simulink model "CR_quarter_car_NL"  (R2025b)
settings: Solver=VariableStepAuto  StartTime=0.0  StopTime=20  RelTol=1e-9
values from neighbouring files (symbols this model uses):
  omega_n1 = 80    [A_quarter_car_parameters.m]    (also in A_uncertain_Plant.m = parameters.omega_n1; Incert_plant.m; LQG.m; LQG_pt2.m)
  tau_1 = 0.005    [A_quarter_car_parameters.m]    (also in LQG.m; LQG_pt2.m; LQG_pt2.mat; Lin_model.m)
  tau_2 = 0.010    (= 0.01)    [A_quarter_car_parameters.m]    (also in LQG.m; LQG_pt2.m; LQG_pt2.mat; Lin_model.m)
  tau_a = 0.025    [A_quarter_car_parameters.m]    (also in A_uncertain_Plant.m = parameters.tau_a; Incert_plant.m; LQG.m; LQG_pt2.m)
  x0_delta_s = 0    [A_quarter_car_parameters.m]    (also in quarter_car_parameters.m)
  x0_delta_t = 0    [A_quarter_car_parameters.m]    (also in quarter_car_parameters.m)
  x0_zs_dot = 0    [A_quarter_car_parameters.m]    (also in quarter_car_parameters.m)
  x0_zu_dot = 0    [A_quarter_car_parameters.m]    (also in quarter_car_parameters.m)
  zeta_1 = 0.7    [A_quarter_car_parameters.m]    (also in A_uncertain_Plant.m = parameters.zeta_1; Incert_plant.m; LQG.m; LQG_pt2.m)
libraries: simulink x12, cstblocks x2
settings Model: Creator=roly2  LastModifiedBy=ettor

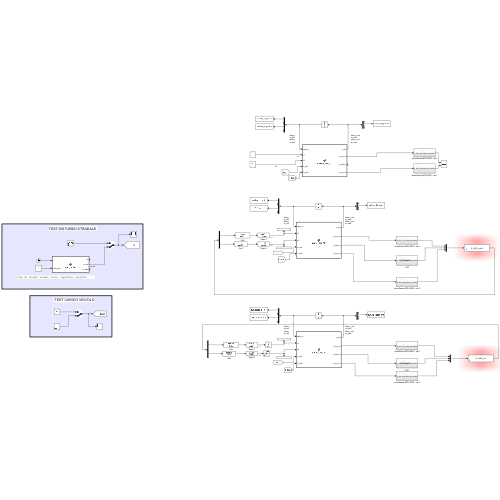
[thumbnail: Simulink's stored preview of the top-level diagram]
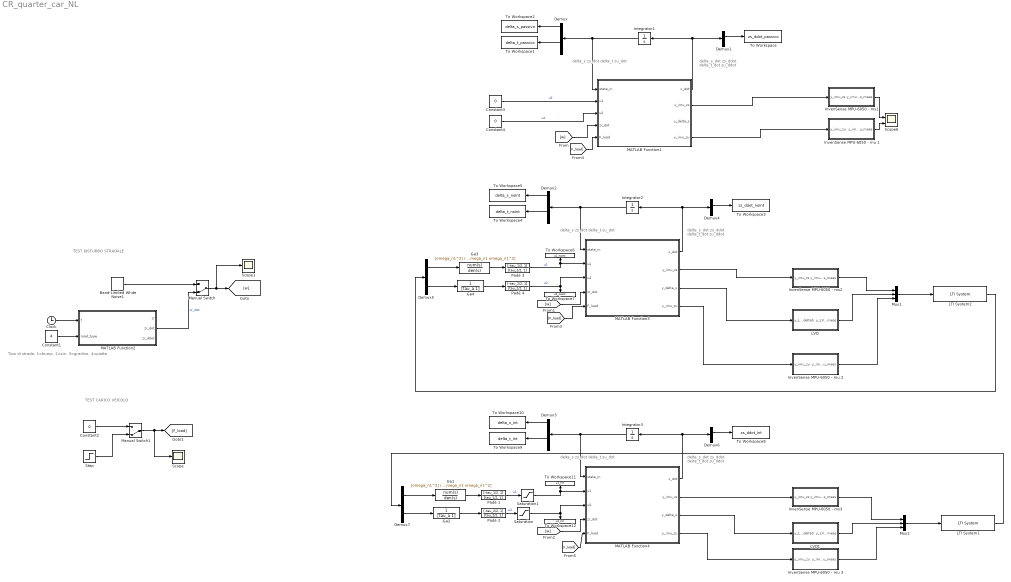
== system CR_quarter_car_NL ==
  note: TEST CARICO VEICOLO
  note: Tipo di strada: 1=bump, 2=sin, 3=gradino, 4=piatta
  note: delta_s_dot
      | zs_ddot
      | delta_t_dot
      | zu_ddot
  note: delta_s
      | zs_dot
      | delta_t
      | zu_dot
  note: delta_s
      | zs_dot
      | delta_t
      | zu_dot
  note: delta_s_dot
      | zs_ddot
      | delta_t_dot
      | zu_ddot
  note: delta_s_dot
      | zs_ddot
      | delta_t_dot
      | zu_ddot
  note: delta_s
      | zs_dot
      | delta_t
      | zu_dot
  note: TEST DISTURBO STRADALE
  Band-Limited White Noise1 : simulink/Sources/Band-Limited White Noise  Cov=[0.0001]  Ts=0.01  seed=[23341]
  Clock : Clock
  Constant1 : Constant  Value=4
  Constant2 : Constant  Value=0
  Constant3 : Constant  Value=0
  Constant4 : Constant  Value=0
  Demux{,1..4,6} (6 alike) : Demux
  Demux5 : Demux  Outputs=2
  Demux7 : Demux  Outputs=2
  Ga1 : TransferFcn  Numerator=[omega_n1^2]  Denominator=[1 2*zeta_1*omega_n1 omega_n1^2]
  Ga2 : TransferFcn  Denominator=[tau_a 1]
  Ga3 : TransferFcn  Numerator=[omega_n1^2]  Denominator=[1 2*zeta_1*omega_n1 omega_n1^2]
  Ga4 : TransferFcn  Denominator=[tau_a 1]
  Integrator1 : Integrator  InitialCondition=[x0_delta_s; x0_zs_dot; x0_delta_t; x0_zu_dot]
  Integrator2 : Integrator  InitialCondition=[x0_delta_s; x0_zs_dot; x0_delta_t; x0_zu_dot]
  Integrator3 : Integrator  InitialCondition=[x0_delta_s; x0_zs_dot; x0_delta_t; x0_zu_dot]
  InvenSense MPU-6050 - ms1 : Subsystem
  InvenSense MPU-6050 - ms2 : Subsystem
  InvenSense MPU-6050 - ms3 : Subsystem
  InvenSense MPU-6050 - mu 1 : Subsystem
  InvenSense MPU-6050 - mu 2 : Subsystem
  InvenSense MPU-6050 - mu 3 : Subsystem
  LTI System1 : cstblocks/LTI System  sys=K_LQG_Int  IC=[]  PadeOrder=0
  LTI System2 : cstblocks/LTI System  sys=K_LQG_noInt  IC=[]  PadeOrder=0
  LVD : Subsystem
  LVD1 : Subsystem
  MATLAB Function1 : MATLAB Function  TreatAsAtomicUnit=on
  MATLAB Function2 : MATLAB Function  TreatAsAtomicUnit=on
  MATLAB Function3 : MATLAB Function  TreatAsAtomicUnit=on
  MATLAB Function4 : MATLAB Function  TreatAsAtomicUnit=on
  Manual Switch : ManualSwitch  CurrentSetting=0
  Manual Switch1 : ManualSwitch  CurrentSetting=0
  Mux1 : Mux  Inputs=3
  Mux2 : Mux  Inputs=3
  Padè 1 : TransferFcn  Numerator=[-tau_1/2, 1]  Denominator=[tau_1/2, 1]
  Padè 2 : TransferFcn  Numerator=[-tau_2/2, 1]  Denominator=[tau_2/2, 1]
  Padè 3 : TransferFcn  Numerator=[-tau_1/2, 1]  Denominator=[tau_1/2, 1]
  Padè 4 : TransferFcn  Numerator=[-tau_2/2, 1]  Denominator=[tau_2/2, 1]
  Saturation : Saturate  UpperLimit=+3000  LowerLimit=-3000
  Saturation1 : Saturate  UpperLimit=+3000  LowerLimit=-3000
  Scope : Scope
      settings: ActiveDisplayYMinimum=-1  ActiveDisplayYMaximum=1
  Scope1 : Scope
  Scope6 : Scope  NumInputPorts=2
      settings: ActiveDisplayYMinimum=-2.689656901745356  ActiveDisplayYMaximum=2.989372585081127  DataLoggingVariableName=ScopeData16
  Step : Step  Time=2  After=500  SampleTime=0
  To Workspace : ToWorkspace  VariableName=zs_ddot_passivo  SaveFormat=Timeseries  SampleTime=-1
  To Workspace1 : ToWorkspace  VariableName=delta_t_passivo  SaveFormat=Timeseries  SampleTime=-1
  To Workspace10 : ToWorkspace  VariableName=delta_s_Int  SaveFormat=Timeseries  SampleTime=-1
  To Workspace11 : ToWorkspace  VariableName=u1_Int  SaveFormat=Timeseries  SampleTime=-1
  To Workspace12 : ToWorkspace  VariableName=u2_Int  SaveFormat=Timeseries  SampleTime=-1
  To Workspace2 : ToWorkspace  VariableName=delta_s_passivo  SaveFormat=Timeseries  SampleTime=-1
  To Workspace3 : ToWorkspace  VariableName=zs_ddot_noInt  SaveFormat=Timeseries  SampleTime=-1
  To Workspace4 : ToWorkspace  VariableName=delta_t_noInt  SaveFormat=Timeseries  SampleTime=-1
  To Workspace5 : ToWorkspace  VariableName=delta_s_noInt  SaveFormat=Timeseries  SampleTime=-1
  To Workspace6 : ToWorkspace  VariableName=u1_noInt  SaveFormat=Timeseries  SampleTime=-1
  To Workspace7 : ToWorkspace  VariableName=u2_noInt  SaveFormat=Timeseries  SampleTime=-1
  To Workspace8 : ToWorkspace  VariableName=zs_ddot_Int  SaveFormat=Timeseries  SampleTime=-1
  To Workspace9 : ToWorkspace  VariableName=delta_t_Int  SaveFormat=Timeseries  SampleTime=-1
  wires:
  Clock/1 -> MATLAB Function2/1(t)
  Constant1/1 -> MATLAB Function2/2(road_type)
  MATLAB Function2/2(zr_dot) -> Manual Switch/2  "zr_dot"
  Band-Limited White Noise1/1 -> Manual Switch/1
  Integrator1/1 -> MATLAB Function1/1(state_in), Demux/1
  MATLAB Function1/4(y_imu_zu) -> InvenSense MPU-6050 - mu 1/1(y_imu_zu)
  MATLAB Function1/2(y_imu_zs) -> InvenSense MPU-6050 - ms1/1(y_imu_zs)
  Constant3/1 -> MATLAB Function1/2(u1)  "u1"
  MATLAB Function1/1(x_dot) -> Demux1/1, Integrator1/1
  InvenSense MPU-6050 - mu 1/1(y_imu_zu_meas) -> Scope6/2
  InvenSense MPU-6050 - ms1/1(y_imu_zs_meas) -> Scope6/1
  Constant4/1 -> MATLAB Function1/3(u2)  "u2"
  [w] -> MATLAB Function1/4(zr_dot)
  Demux1/2 -> To Workspace/1
  Demux/3 -> To Workspace1/1
  Demux/1 -> To Workspace2/1
  Demux2/3 -> To Workspace4/1
  Demux2/1 -> To Workspace5/1
  [w] -> MATLAB Function3/4(zr_dot)
  Demux4/2 -> To Workspace3/1
  MATLAB Function3/1(x_dot) -> Demux4/1, Integrator2/1
  Mux1/1 -> LTI System2/1
  MATLAB Function3/4(y_imu_zu) -> InvenSense MPU-6050 - mu 2/1(y_imu_zu)
  Integrator2/1 -> MATLAB Function3/1(state_in), Demux2/1
  MATLAB Function3/2(y_imu_zs) -> InvenSense MPU-6050 - ms2/1(y_imu_zs)
  Ga3/1 -> Padè 3/1
  Ga4/1 -> Padè 4/1
  Padè 3/1 -> To Workspace6/1, MATLAB Function3/2(u1)  "u1"
  Padè 4/1 -> MATLAB Function3/3(u2), To Workspace7/1  "u2"
  Demux5/1 -> Ga3/1
  Demux5/2 -> Ga4/1
  LTI System2/1 -> Demux5/1
  Demux7/2 -> Ga2/1
  Ga2/1 -> Padè 2/1
  Demux3/3 -> To Workspace9/1
  Demux3/1 -> To Workspace10/1
  [w] -> MATLAB Function4/4(zr_dot)
  Integrator3/1 -> MATLAB Function4/1(state_in), Demux3/1
  Demux7/1 -> Ga1/1
  MATLAB Function4/2(y_imu_zs) -> InvenSense MPU-6050 - ms3/1(y_imu_zs)
  Ga1/1 -> Padè 1/1
  Mux2/1 -> LTI System1/1
  Demux6/2 -> To Workspace8/1
  Padè 2/1 -> Saturation/1  "u2"
  MATLAB Function4/1(x_dot) -> Demux6/1, Integrator3/1
  LTI System1/1 -> Demux7/1
  Padè 1/1 -> Saturation1/1  "u1"
  MATLAB Function4/4(y_imu_zu) -> InvenSense MPU-6050 - mu 3/1(y_imu_zu)
  InvenSense MPU-6050 - ms2/1(y_imu_zs_meas) -> Mux1/1
  InvenSense MPU-6050 - mu 2/1(y_imu_zu_meas) -> Mux1/3
  InvenSense MPU-6050 - ms3/1(y_imu_zs_meas) -> Mux2/1
  InvenSense MPU-6050 - mu 3/1(y_imu_zu_meas) -> Mux2/3
  [F_load] -> MATLAB Function3/5(F_load)
  [F_load] -> MATLAB Function1/5(F_load)
  [F_load] -> MATLAB Function4/5(F_load)
  MATLAB Function3/3(y_delta_s) -> LVD/1(y_LVDT_deltaS)
  LVD/1(y_LVDT_deltaS_meas) -> Mux1/2
  MATLAB Function4/3(y_delta_s) -> LVD1/1(y_LVDT_deltaS)
  Saturation/1 -> MATLAB Function4/3(u2), To Workspace12/1
  Saturation1/1 -> To Workspace11/1, MATLAB Function4/2(u1)
  LVD1/1(y_LVDT_deltaS_meas) -> Mux2/2
  Constant2/1 -> Manual Switch1/1
  Step/1 -> Manual Switch1/2
  Manual Switch1/1 -> Scope/1, [F_load]
  Manual Switch/1 -> Scope1/1, [w]

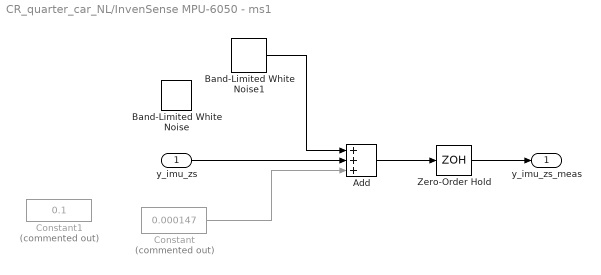
== system CR_quarter_car_NL/InvenSense MPU-6050 - ms1 ==
  y_imu_zs : Inport
  Add : Sum  Inputs=+++
  Band-Limited White Noise : simulink/Sources/Band-Limited White Noise  Cov=[3.5*10^-7]  Ts=0.01  seed=[1234]
  Band-Limited White Noise1 : simulink/Sources/Band-Limited White Noise  Cov=0.0001  Ts=0.01  seed=[1234]
  Constant : Constant  Commented=on  Value=0.000147
  Constant1 : Constant  Commented=on  Value=0.1
  Zero-Order Hold : ZeroOrderHold  SampleTime=0.01
  y_imu_zs_meas : Outport
  wires:
  Add/1 -> Zero-Order Hold/1
  y_imu_zs/1 -> Add/2
  Constant/1 -> Add/3
  Zero-Order Hold/1 -> y_imu_zs_meas/1
  Band-Limited White Noise1/1 -> Add/1

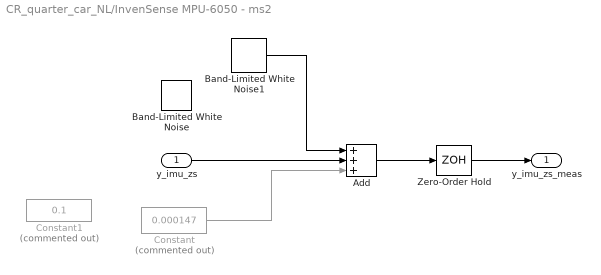
== system CR_quarter_car_NL/InvenSense MPU-6050 - ms2 ==
  y_imu_zs : Inport
  Add : Sum  Inputs=+++
  Band-Limited White Noise : simulink/Sources/Band-Limited White Noise  Cov=[3.5*10^-7]  Ts=0.01  seed=[1234]
  Band-Limited White Noise1 : simulink/Sources/Band-Limited White Noise  Cov=0.0001  Ts=0.01  seed=[1234]
  Constant : Constant  Commented=on  Value=0.000147
  Constant1 : Constant  Commented=on  Value=0.1
  Zero-Order Hold : ZeroOrderHold  SampleTime=0.01
  y_imu_zs_meas : Outport
  wires:
  Add/1 -> Zero-Order Hold/1
  y_imu_zs/1 -> Add/2
  Constant/1 -> Add/3
  Zero-Order Hold/1 -> y_imu_zs_meas/1
  Band-Limited White Noise1/1 -> Add/1

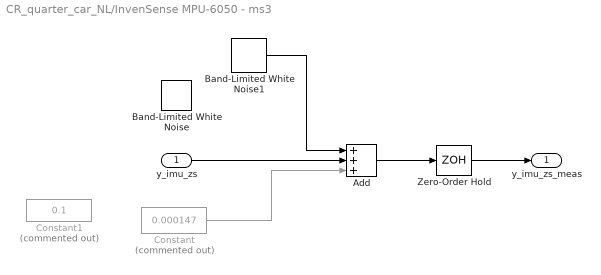
== system CR_quarter_car_NL/InvenSense MPU-6050 - ms3 ==
  y_imu_zs : Inport
  Add : Sum  Inputs=+++
  Band-Limited White Noise : simulink/Sources/Band-Limited White Noise  Cov=[3.5*10^-7]  Ts=0.01  seed=[1234]
  Band-Limited White Noise1 : simulink/Sources/Band-Limited White Noise  Cov=0.0001  Ts=0.01  seed=[1234]
  Constant : Constant  Commented=on  Value=0.000147
  Constant1 : Constant  Commented=on  Value=0.1
  Zero-Order Hold : ZeroOrderHold  SampleTime=0.01
  y_imu_zs_meas : Outport
  wires:
  Add/1 -> Zero-Order Hold/1
  y_imu_zs/1 -> Add/2
  Constant/1 -> Add/3
  Zero-Order Hold/1 -> y_imu_zs_meas/1
  Band-Limited White Noise1/1 -> Add/1

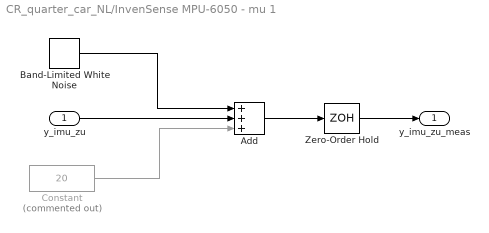
== system CR_quarter_car_NL/InvenSense MPU-6050 - mu 1 ==
  y_imu_zu : Inport
  Add : Sum  Inputs=+++
  Band-Limited White Noise : simulink/Sources/Band-Limited White Noise  Cov=0.0002  Ts=0.02  seed=[23341]
  Constant : Constant  Commented=on  Value=20
  Zero-Order Hold : ZeroOrderHold  SampleTime=0.02
  y_imu_zu_meas : Outport
  wires:
  Add/1 -> Zero-Order Hold/1
  y_imu_zu/1 -> Add/2
  Constant/1 -> Add/3
  Band-Limited White Noise/1 -> Add/1
  Zero-Order Hold/1 -> y_imu_zu_meas/1

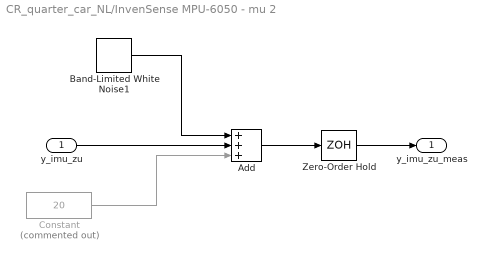
== system CR_quarter_car_NL/InvenSense MPU-6050 - mu 2 ==
  y_imu_zu : Inport
  Add : Sum  Inputs=+++
  Band-Limited White Noise1 : simulink/Sources/Band-Limited White Noise  Cov=0.0001  Ts=0.01  seed=[1234]
  Constant : Constant  Commented=on  Value=20
  Zero-Order Hold : ZeroOrderHold  SampleTime=0.01
  y_imu_zu_meas : Outport
  wires:
  Add/1 -> Zero-Order Hold/1
  y_imu_zu/1 -> Add/2
  Constant/1 -> Add/3
  Zero-Order Hold/1 -> y_imu_zu_meas/1
  Band-Limited White Noise1/1 -> Add/1

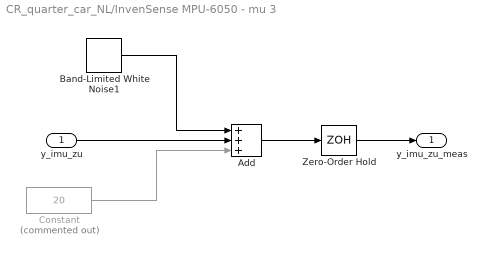
== system CR_quarter_car_NL/InvenSense MPU-6050 - mu 3 ==
  y_imu_zu : Inport
  Add : Sum  Inputs=+++
  Band-Limited White Noise1 : simulink/Sources/Band-Limited White Noise  Cov=0.0001  Ts=0.01  seed=[1234]
  Constant : Constant  Commented=on  Value=20
  Zero-Order Hold : ZeroOrderHold  SampleTime=0.01
  y_imu_zu_meas : Outport
  wires:
  Add/1 -> Zero-Order Hold/1
  y_imu_zu/1 -> Add/2
  Constant/1 -> Add/3
  Zero-Order Hold/1 -> y_imu_zu_meas/1
  Band-Limited White Noise1/1 -> Add/1

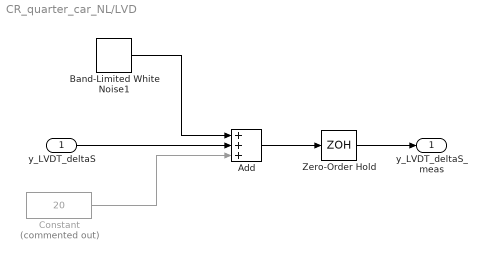
== system CR_quarter_car_NL/LVD ==
  y_LVDT_deltaS : Inport
  Add : Sum  Inputs=+++
  Band-Limited White Noise1 : simulink/Sources/Band-Limited White Noise  Cov=1e-8  Ts=0.01  seed=[4567]
  Constant : Constant  Commented=on  Value=20
  Zero-Order Hold : ZeroOrderHold  SampleTime=0.01
  y_LVDT_deltaS_meas : Outport
  wires:
  Add/1 -> Zero-Order Hold/1
  y_LVDT_deltaS/1 -> Add/2
  Constant/1 -> Add/3
  Zero-Order Hold/1 -> y_LVDT_deltaS_meas/1
  Band-Limited White Noise1/1 -> Add/1

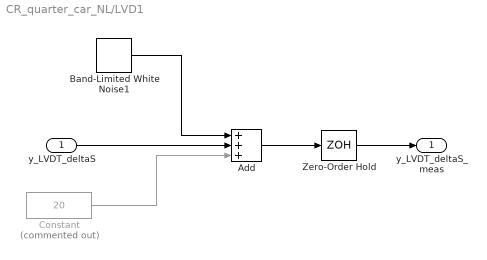
== system CR_quarter_car_NL/LVD1 ==
  y_LVDT_deltaS : Inport
  Add : Sum  Inputs=+++
  Band-Limited White Noise1 : simulink/Sources/Band-Limited White Noise  Cov=1e-8  Ts=0.01  seed=[4567]
  Constant : Constant  Commented=on  Value=20
  Zero-Order Hold : ZeroOrderHold  SampleTime=0.01
  y_LVDT_deltaS_meas : Outport
  wires:
  Add/1 -> Zero-Order Hold/1
  y_LVDT_deltaS/1 -> Add/2
  Constant/1 -> Add/3
  Zero-Order Hold/1 -> y_LVDT_deltaS_meas/1
  Band-Limited White Noise1/1 -> Add/1

== matlab function CR_quarter_car_NL/MATLAB Function1 ==
  data: state_in input; x_dot output; u1 input; u2 input; zr_dot input; F_load input; parameters parameter; y_imu_zs output; y_delta_s output; y_imu_zu output
function [x_dot,y_imu_zs, y_delta_s , y_imu_zu ] = quarter_car_NL(state_in, u1, u2, zr_dot, F_load ,parameters)

    delta_s = state_in(1);
    zs_dot = state_in(2);
    delta_t = state_in(3);
    zu_dot = state_in(4);
    
    m_s = parameters.m_s;
    m_u = parameters.m_u;
    ks0 = parameters.ks0;
    alpha = parameters.alpha;
    bs = parameters.bs;
    kt = parameters.kt;
    bt = parameters.bt;
    
    delta_s_dot = zs_dot - zu_dot;
    delta_t_dot = zu_dot - zr_dot;
    
    Fs = ks0 * delta_s + alpha * delta_s^3 + bs * delta_s_dot;
    Ft = kt * delta_t + bt * delta_t_dot;
    
    
    zs_ddot = (-Fs + u1-F_load) / m_s;
    zu_ddot = (Fs - Ft - u1 + u2) / m_u;
    
    x_dot = [delta_s_dot; zs_ddot; delta_t_dot; zu_ddot];
    
    y_imu_zs = zs_ddot; 
    y_imu_zu = zu_ddot;
    y_delta_s = delta_s; % Sensore di altezza (Ride Height) 

end

== matlab function CR_quarter_car_NL/MATLAB Function4 ==
  data: state_in input; x_dot output; u1 input; u2 input; zr_dot input; F_load input; parameters parameter; y_imu_zs output; y_delta_s output; y_imu_zu output
function [x_dot,y_imu_zs, y_delta_s , y_imu_zu ] = quarter_car_NL(state_in, u1, u2, zr_dot, F_load ,parameters)

    delta_s = state_in(1);
    zs_dot = state_in(2);
    delta_t = state_in(3);
    zu_dot = state_in(4);
    
    m_s = parameters.m_s;
    m_u = parameters.m_u;
    ks0 = parameters.ks0;
    alpha = parameters.alpha;
    bs = parameters.bs;
    kt = parameters.kt;
    bt = parameters.bt;
    
    delta_s_dot = zs_dot - zu_dot;
    delta_t_dot = zu_dot - zr_dot;
    
    Fs = ks0 * delta_s + alpha * delta_s^3 + bs * delta_s_dot;
    Ft = kt * delta_t + bt * delta_t_dot;
    
    
    zs_ddot = (-Fs + u1-F_load) / m_s;
    zu_ddot = (Fs - Ft - u1 + u2) / m_u;
    
    x_dot = [delta_s_dot; zs_ddot; delta_t_dot; zu_ddot];
    
    y_imu_zs = zs_ddot; 
    y_imu_zu = zu_ddot;
    y_delta_s = delta_s; % Sensore di altezza (Ride Height) 

end

== matlab function CR_quarter_car_NL/MATLAB Function2 ==
  data: t input; zr output; zr_dot output; zr_ddot output; params parameter; road_type input
function [zr, zr_dot, zr_ddot] = road_profile(t, params, road_type)
%   road_type = 1 bump | 2 sinusoide | 3 gradino | 4 piatta

    switch road_type
        case 1  % ---- BUMP ----

            A = params.A;   % altezza [m]
            L = params.L;   % lunghezza [m]
            v = params.v;   % velocità veicolo [m/s]
            t0 = params.t0; % istante di inizio ostacolo [s]
            T = L / v;      % durata temporale bump
            
            % Il dosso inizia a t0 e finisce a t0 + T
            if t >= t0 && t <= (t0 + T)
                t_rel = t - t0; % Tempo relativo (parte da 0 quando inizia il dosso)
                phi   = 2*pi*v*t_rel / L;
                zr    = (A/2) * (1 - cos(phi));
                zr_dot   = (A*pi*v/L) * sin(phi);
                zr_ddot  = (A*2*pi^2*v^2/L^2) * cos(phi);
            else
                zr = 0;  zr_dot = 0;  zr_ddot = 0;
            end
            
        case 2  % ---- SINUSOIDE ----
            A = params.A;   % ampiezza [m]
            f = params.f;   % frequenza [Hz]
            t0 = params.t0; % istante di inizio ostacolo [s]
            
            % La strada vibra solo dopo t0
            if t >= t0
                t_rel = t - t0; % Tempo relativo
                w = 2*pi*f;
                zr   =  A * sin(w*t_rel);
                zr_dot  =  A * w * cos(w*t_rel);
                zr_ddot = -A * w^2 * sin(w*t_rel);
            else
                zr = 0;  zr_dot = 0;  zr_ddot = 0;
            end
            
        case 3  % ---- GRADINO SMUSSATO ----
            A  = params.A;    % altezza [m]
            t0 = params.t0;   % istante del gradino [s]
            tau = params.tau/1000; % tempo di salita [s]
            
            arg  = (t - t0) / tau;
            zr   = (A/2) * (1 + tanh(arg));
            zr_dot  = (A/(2*tau)) * (sech(arg))^2;
            zr_ddot = -(A/tau^2) * (sech(arg))^2 * tanh(arg);
            
        case 4  % ---- STRADA PIATTA ----
            zr = 0;  zr_dot = 0;  zr_ddot = 0;
            
        otherwise 
            zr = 0;  zr_dot = 0;  zr_ddot = 0;
    end
end

== matlab function CR_quarter_car_NL/MATLAB Function3 ==
  data: state_in input; x_dot output; u1 input; u2 input; zr_dot input; F_load input; parameters parameter; y_imu_zs output; y_delta_s output; y_imu_zu output
function [x_dot,y_imu_zs, y_delta_s , y_imu_zu ] = quarter_car_NL(state_in, u1, u2, zr_dot, F_load ,parameters)

    delta_s = state_in(1);
    zs_dot = state_in(2);
    delta_t = state_in(3);
    zu_dot = state_in(4);
    
    m_s = parameters.m_s;
    m_u = parameters.m_u;
    ks0 = parameters.ks0;
    alpha = parameters.alpha;
    bs = parameters.bs;
    kt = parameters.kt;
    bt = parameters.bt;
    
    delta_s_dot = zs_dot - zu_dot;
    delta_t_dot = zu_dot - zr_dot;
    
    Fs = ks0 * delta_s + alpha * delta_s^3 + bs * delta_s_dot;
    Ft = kt * delta_t + bt * delta_t_dot;
    
    
    zs_ddot = (-Fs + u1-F_load) / m_s;
    zu_ddot = (Fs - Ft - u1 + u2) / m_u;
    
    x_dot = [delta_s_dot; zs_ddot; delta_t_dot; zu_ddot];
    
    y_imu_zs = zs_ddot; 
    y_imu_zu = zu_ddot;
    y_delta_s = delta_s; % Sensore di altezza (Ride Height) 

end
